simulink subsystem "Motor"  (R2021b)
settings: Solver=VariableStepAuto  StartTime=0.0  StopTime=10.0  RelTol=1e-3
undefined symbols (not defined in the file): Angle, Current, Speed, Ts_Curr, x607325_CurrMinA, x607325_Res, x607325_RotIner, x607325_VNom
libraries: fl_lib x5, nesl_utility x2, ee_lib x1
settings Model: Creator=khoi  LastModifiedBy=khoi
settings SolverCC: AlgebraicLoopSolver=TrustRegion
settings DebuggingCC: SFMachineParentedDataDiag=warning

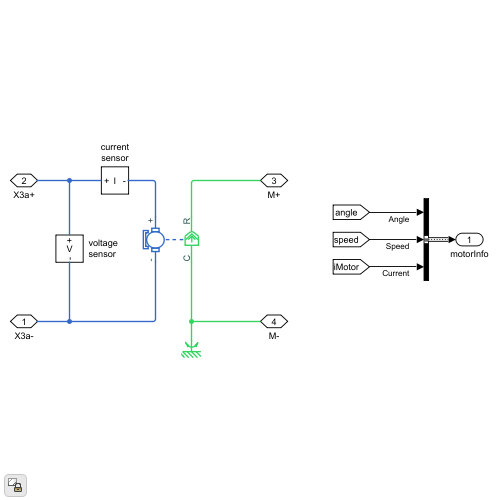
[thumbnail: Simulink's stored preview of the top-level diagram]
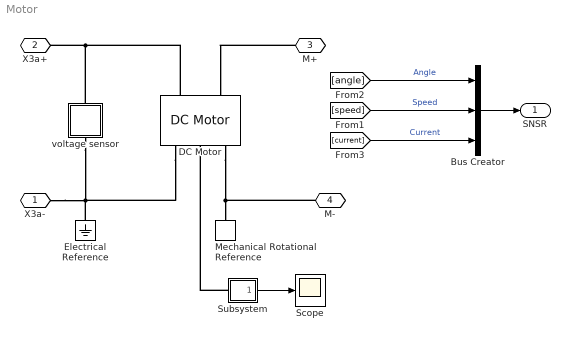
== system Motor ==
  Bus Creator : BusCreator  Inputs=Angle,Speed,Current  OutDataTypeStr=Bus: motorInfo  NonVirtualBus=on
  DC Motor : ee_lib/Electromechanical/Brushed Motors/DC Motor  field_option=ee.enum.field_option.pm  Rf=100 Ohm  Lf=1 H  Laf=0.15 H  If0=0 A  parameterization=ee.enum.dcparam_option.torque_speed  Ra=3.9 Ohm  La=x607325_RotInd mH  emf_or_torque=ee.enum.emf_or_torque.kv  Kv=0.072e-3 V/rpm  Ki=6.876e-4 N*m/A  T_stall=x607325_TorqMax mN*m  w_max=x607325_RotOmgMax rpm  w_rated=Speed rpm  P_rated=0.08 W  V_rated=x607325_VNom V  lam_param=ee.enum.lam_param.current  i_noload=x607325_CurrMinA A  V_i_noload=x607325_VNom-x607325_Res*x607325_CurrMinA V  J=x607325_RotIner g*cm^2  lam=0 N*m/(rad/s)  speed0=0 rpm  enable_fault_armature=simscape.enum.onoff.off  rev_faulted=1/2  G_faulted_armature=1e-3 S  fault_trigger_armature=ee.enum.faults.faultTrigger.temporal  t_fault_armature=1 s  max_permissible_current_armature=inf A  t_fail_on_current_armature=1 s  enable_fault_field=simscape.enum.onoff.off  G_faulted_field=1e-5 S  fault_trigger_field=ee.enum.faults.faultTrigger.temporal  t_fault_field=1 s  max_permissible_current_field=inf A  t_fail_on_current_field=1 s  fault_action=simscape.enum.assert.action.warn  alpha=3.93e-3 1/K  Tmeas=25 degC  thermal_mass=100 J/K  initial_temperature=25 degC
      settings: InternalSimscapePortConfiguration="{\"Bottom\":[],\"Left\":[{\"id\":\"p\",\"label\":\"+\",\"type\":\"foundation.electrical.electrical\"},{\"id\":\"R\",\"label\":\"R\",\"type\":\"foundation.mechanical.rotational.rotational\"}],\"Right\":[{\"id\":\"n\",\"label\":\"-\",\"type\":\"foundation.electrical.electrical\"},{\"id\":\"H\",\"label\":\"H\",\"type\":\"foundation.thermal.thermal\"},{\"id\":\"C\",\"label\":\"C\",\"type\":\"foundation.mechanical.rotational.rotational\"}],\"Top\":[]}"
  Electrical Reference : fl_lib/Electrical/Electrical Elements/Electrical Reference
  Mechanical Rotational Reference : fl_lib/Mechanical/Rotational Elements/Mechanical Rotational Reference
  Scope : Scope
  Subsystem : Subsystem
  voltage sensor : Subsystem
      mask Display: disp('V')
  X3a- : PMIOPort  Side=Left
  X3a+ : PMIOPort  Port=2  Side=Left
  M+ : PMIOPort  Port=3  Side=Left
  M- : PMIOPort  Port=4  Side=Left
  SNSR : Outport
  wires:
  [current] -> Bus Creator/3  "Current"
  [angle] -> Bus Creator/1  "Angle"
  [speed] -> Bus Creator/2  "Speed"
  Bus Creator/1 -> SNSR/1
  Subsystem/1(Out1) -> Scope/1
  connections:
  M-/RConn1 -- Mechanical Rotational Reference/LConn1 -- DC Motor/RConn3
  Electrical Reference/LConn1 -- X3a-/RConn1 -- DC Motor/RConn1 -- voltage sensor/RConn1
  DC Motor/LConn1 -- X3a+/RConn1 -- voltage sensor/LConn1
  Subsystem/LConn1 -- DC Motor/RConn2
  M+/RConn1 -- DC Motor/LConn2

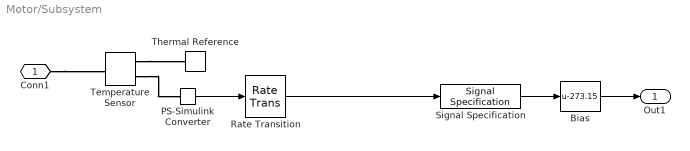
== system Motor/Subsystem ==
  Bias : Bias  Bias=-273.15
  PS-Simulink Converter : nesl_utility/PS-Simulink Converter  PhysicalDomain=network_engine_domain  SubClassName=ps_output  LeftPortType=input  RightPortType=output  PseudoPeriodic=off  Frequencies=[]  Unit=inherit  AffineConversion=on
      settings: SourceProductBaseCode=PW,SS
  Rate Transition : RateTransition
  Signal Specification : SignalSpecification  SampleTime=Ts_Curr
  Temperature Sensor : fl_lib/Thermal/Thermal Sensors/Temperature Sensor
  Thermal Reference : fl_lib/Thermal/Thermal Elements/Thermal Reference
  Conn1 : PMIOPort  Side=Left
  Out1 : Outport
  wires:
  Rate Transition/1 -> Signal Specification/1
  PS-Simulink Converter/1 -> Rate Transition/1
  Bias/1 -> Out1/1
  Signal Specification/1 -> Bias/1
  connections:
  Conn1/RConn1 -- Temperature Sensor/LConn1
  Temperature Sensor/RConn2 -- PS-Simulink Converter/LConn1
  Temperature Sensor/RConn1 -- Thermal Reference/LConn1

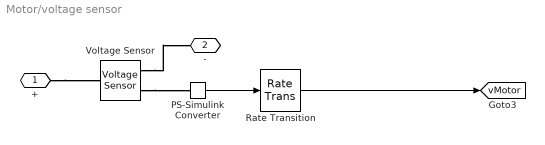
== system Motor/voltage sensor ==
  PS-Simulink Converter : nesl_utility/PS-Simulink Converter  PhysicalDomain=network_engine_domain  SubClassName=ps_output  LeftPortType=input  RightPortType=output  PseudoPeriodic=off  Frequencies=[]  Unit=inherit  AffineConversion=off
      settings: SourceProductBaseCode=PW,SS
  Rate Transition : RateTransition
  Voltage Sensor : fl_lib/Electrical/Electrical Sensors/Voltage Sensor
  + : PMIOPort  Side=Left
  - : PMIOPort  Port=2  Side=Right
  tag scope: vMotor=global
  wires:
  Rate Transition/1 -> [vMotor]
  PS-Simulink Converter/1 -> Rate Transition/1
  connections:
  Voltage Sensor/RConn2 -- -/RConn1
  +/RConn1 -- Voltage Sensor/LConn1
  Voltage Sensor/RConn1 -- PS-Simulink Converter/LConn1
